simulink model "dgbe_test"  (Simulink 7.4)
settings: Solver=ode45  StartTime=0.0  StopTime=10.0  RelTol=1e-3
undefined symbols (not defined in the file or in its folder): ROACH
libraries: xbsIndex_r4 x109, xps_library x27
settings Model: Creator=tfiliba  LastModifiedBy=tfiliba

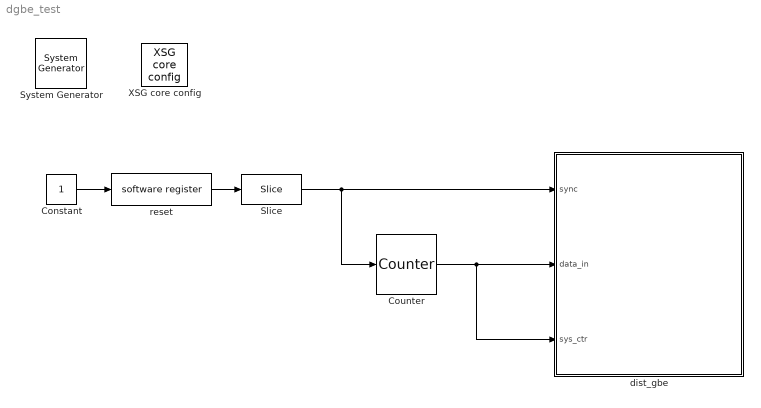
== system dgbe_test ==
  " System Generator" : xbsIndex_r4/ System Generator  Tag=genX  SystemSampleTime=-1  xilinxfamily=virtex5  part=xc5vsx95t  speed=-1  package=ff1136  synthesis_tool=XST  clock_wrapper=Clock Enables  directory=./dgbe_test/sysgen  testbench=off  simulink_period=1  sysclk_period=3.9062  dcm_input_clock_period=100  incr_netlist=off  trim_vbits=Everywhere in SubSystem  dbl_ovrd=According to Block Masks  core_generation=According to Block Masks  run_coregen=off  deprecated_control=off  eval_field=0  block_type=sysgen
      settings: block_version=11.4
  Constant : Constant  OutDataType=fixdt(1, 16)  OutScaling=2^0
  Counter : xbsIndex_r4/Counter  cnt_type=Free Running  cnt_to=Inf  operation=Up  start_count=0  cnt_by_val=1  arith_type=Unsigned  n_bits=64  bin_pt=0  load_pin=off  rst=on  en=off  explicit_period=on  period=1  dbl_ovrd=off  use_behavioral_HDL=off  implementation=Fabric  block_type=counter
      settings: block_version=11.4
  Slice : xbsIndex_r4/Slice  nbits=1  boolean_output=on  mode=Upper Bit Location + Width  bit1=0  base1=MSB of Input  bit0=0  base0=LSB of Input  dbl_ovrd=off  block_type=slice
  XSG core config : xps_library/XSG core config  Tag=xps:xsg  SystemSampleTime=-1  hw_sys=ROACH:sx95t  ibob_linux=off  clk_src=aux0_clk  iBOB_clk_src=sys_clk  BEE2_ctrl_clk_src=sys_clk  BEE2_usr_clk_src=sys_clk  ROACH_clk_src=aux0_clk  CORR_clk_src=sys_clk  gpio_clk_io_group=iBOB:sma  gpio_clk_bit_index=0  clk_rate=256  sample_period=1  synthesis_tool=XST  mpc_type=powerpc440_ext
  dist_gbe : Subsystem  mask(dist_gbe){numcomputers=8, samplesperpacket=1024, numtengbe=4}
      mask prompts: numcomputers "Num IPs (Must be power of 2)"; samplesperpacket "Samples per packet (Number of samples to put in a packet)"; numtengbe "Number of tengbe ports"
      mask init:
      | cfg.source = str2func('dist_gbe_xblock_init');
      | cfg.toplevel = gcb;
      | cfg.depend = {'dist_gbe_xblock_init.m'};
      | args = {numcomputers,samplesperpacket,numtengbe};
      | xBlock(cfg, args);
  reset : xps_library/software register  Tag=xps:sw_reg  SystemSampleTime=-1  io_dir=From Processor  arith_type=Unsigned  bitwidth=32  bin_pt=0  sample_period=1  gw_name=dgbe_test_reset_user_data_out
  wires:
  Constant/1 -> reset/1
  Counter/1 -> dist_gbe/2(data_in), dist_gbe/3(sys_ctr)
  reset/1 -> Slice/1
  Slice/1 -> Counter/1, dist_gbe/1(sync)

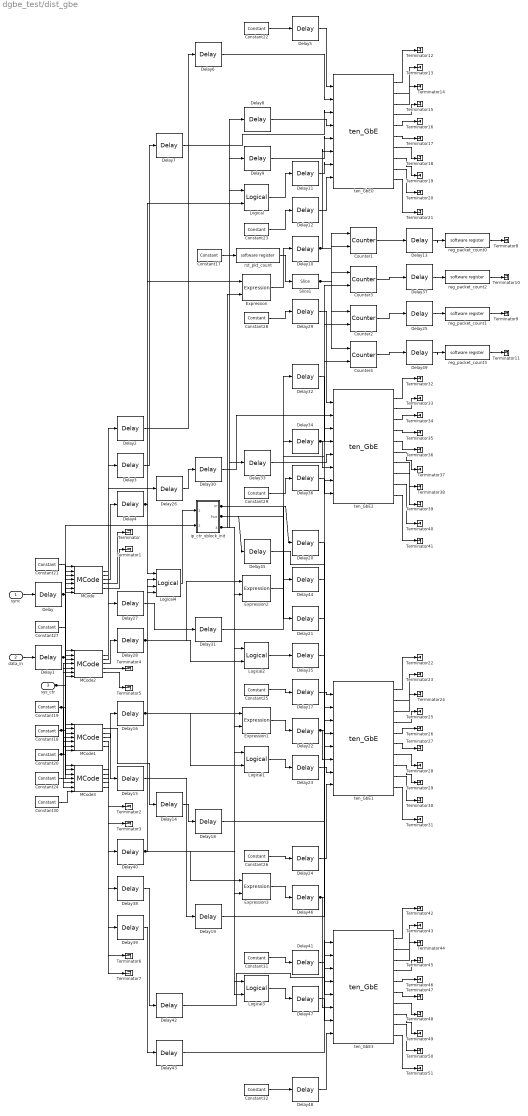
== system dgbe_test/dist_gbe ==
  sync : Inport
  data_in : Inport  Port=2
  sys_ctr : Inport  Port=3
  Constant17 : xbsIndex_r4/Constant  arith_type=Signed (2's comp)  const=0  n_bits=16  bin_pt=14  explicit_period=on  period=1  equ=P=C  opselect=C  inp2=PCIN>>17  opr=+  inp1=P  carry=CIN  dbl_ovrd=off  block_type=constant
      settings: block_version=11.4
  Constant18 : xbsIndex_r4/Constant  arith_type=Signed (2's comp)  const=8  n_bits=4  bin_pt=0  explicit_period=on  period=1  equ=P=C  opselect=C  inp2=PCIN>>17  opr=+  inp1=P  carry=CIN  dbl_ovrd=off  block_type=constant
      settings: block_version=11.4
  Constant19 : xbsIndex_r4/Constant  arith_type=Signed (2's comp)  const=1024  n_bits=11  bin_pt=0  explicit_period=on  period=1  equ=P=C  opselect=C  inp2=PCIN>>17  opr=+  inp1=P  carry=CIN  dbl_ovrd=off  block_type=constant
      settings: block_version=11.4
  Constant20 : xbsIndex_r4/Constant  arith_type=Signed (2's comp)  const=4  n_bits=3  bin_pt=0  explicit_period=on  period=1  equ=P=C  opselect=C  inp2=PCIN>>17  opr=+  inp1=P  carry=CIN  dbl_ovrd=off  block_type=constant
      settings: block_version=11.4
  Constant21 : xbsIndex_r4/Constant  arith_type=Signed (2's comp)  const=0  n_bits=3  bin_pt=0  explicit_period=on  period=1  equ=P=C  opselect=C  inp2=PCIN>>17  opr=+  inp1=P  carry=CIN  dbl_ovrd=off  block_type=constant
      settings: block_version=11.4
  Constant{22..23,25..26,28..29,31..32} (8 alike) : xbsIndex_r4/Constant  arith_type=Boolean  const=0  n_bits=16  bin_pt=14  explicit_period=on  period=1  equ=P=C  opselect=C  inp2=PCIN>>17  opr=+  inp1=P  carry=CIN  dbl_ovrd=off  block_type=constant
      settings: block_version=11.4
  Constant24 : xbsIndex_r4/Constant  arith_type=Signed (2's comp)  const=1  n_bits=3  bin_pt=0  explicit_period=on  period=1  equ=P=C  opselect=C  inp2=PCIN>>17  opr=+  inp1=P  carry=CIN  dbl_ovrd=off  block_type=constant
      settings: block_version=11.4
  Constant27 : xbsIndex_r4/Constant  arith_type=Signed (2's comp)  const=2  n_bits=3  bin_pt=0  explicit_period=on  period=1  equ=P=C  opselect=C  inp2=PCIN>>17  opr=+  inp1=P  carry=CIN  dbl_ovrd=off  block_type=constant
      settings: block_version=11.4
  Constant30 : xbsIndex_r4/Constant  arith_type=Signed (2's comp)  const=3  n_bits=3  bin_pt=0  explicit_period=on  period=1  equ=P=C  opselect=C  inp2=PCIN>>17  opr=+  inp1=P  carry=CIN  dbl_ovrd=off  block_type=constant
      settings: block_version=11.4
  Counter{1..4} (4 alike) : xbsIndex_r4/Counter  cnt_type=Free Running  cnt_to=Inf  operation=Up  start_count=0  cnt_by_val=1  arith_type=Unsigned  n_bits=32  bin_pt=0  load_pin=off  rst=on  en=on  explicit_period=on  period=1  dbl_ovrd=off  use_behavioral_HDL=off  implementation=Fabric  block_type=counter
      settings: block_version=11.4
  Delay : xbsIndex_r4/Delay  en=off  latency=3  dbl_ovrd=off  reg_retiming=on  block_type=delay
      settings: block_version=11.4
  Delay1 : xbsIndex_r4/Delay  en=off  latency=3  dbl_ovrd=off  reg_retiming=on  block_type=delay
      settings: block_version=11.4
  Delay{2..49} (48 alike) : xbsIndex_r4/Delay  en=off  latency=2  dbl_ovrd=off  reg_retiming=on  block_type=delay
      settings: block_version=11.4
  Expression{,1..3} (4 alike) : xbsIndex_r4/Expression  expression=a&~b  align_bp=on  en=off  latency=0  precision=Full  arith_type=Unsigned  n_bits=16  bin_pt=0  dbl_ovrd=off  block_type=expr
      settings: block_version=11.4
  Logical{,1..3} (4 alike) : xbsIndex_r4/Logical  logical_function=AND  inputs=2  en=off  latency=0  precision=Full  arith_type=Unsigned  n_bits=16  bin_pt=0  align_bp=on  dbl_ovrd=off  block_type=logical
      settings: block_version=11.4
  Logical4 : xbsIndex_r4/Logical  logical_function=OR  inputs=4  en=off  latency=0  precision=Full  arith_type=Unsigned  n_bits=16  bin_pt=0  align_bp=on  dbl_ovrd=off  block_type=logical
      settings: block_version=11.4
  MCode{,1..3} (4 alike) : xbsIndex_r4/MCode  mfname=packetizer.m  explicit_period=off  period=1  dbl_ovrd=off  enable_stdout=off  enable_debug=off  suppress_output=on  defparams={}  hide_port_list={}  block_type=mcode
      settings: block_version=11.4
  Slice1 : xbsIndex_r4/Slice  nbits=1  boolean_output=on  mode=Upper Bit Location + Width  bit1=0  base1=MSB of Input  bit0=0  base0=LSB of Input  dbl_ovrd=off  block_type=slice
  Terminator{,1..51} (52 alike) : Terminator
  ip_ctr_xblock_init : Subsystem
  reg_packet_count0 : xps_library/software register  Tag=xps:sw_reg  SystemSampleTime=-1  io_dir=To Processor  arith_type=Unsigned  bitwidth=32  bin_pt=0  sample_period=1  gw_name=dgbe_test_dist_gbe_reg_packet_count0_user_data_in
  reg_packet_count1 : xps_library/software register  Tag=xps:sw_reg  SystemSampleTime=-1  io_dir=To Processor  arith_type=Unsigned  bitwidth=32  bin_pt=0  sample_period=1  gw_name=dgbe_test_dist_gbe_reg_packet_count1_user_data_in
  reg_packet_count2 : xps_library/software register  Tag=xps:sw_reg  SystemSampleTime=-1  io_dir=To Processor  arith_type=Unsigned  bitwidth=32  bin_pt=0  sample_period=1  gw_name=dgbe_test_dist_gbe_reg_packet_count2_user_data_in
  reg_packet_count3 : xps_library/software register  Tag=xps:sw_reg  SystemSampleTime=-1  io_dir=To Processor  arith_type=Unsigned  bitwidth=32  bin_pt=0  sample_period=1  gw_name=dgbe_test_dist_gbe_reg_packet_count3_user_data_in
  rst_pkt_count : xps_library/software register  Tag=xps:sw_reg  SystemSampleTime=-1  io_dir=From Processor  arith_type=Unsigned  bitwidth=32  bin_pt=0  sample_period=1  gw_name=dgbe_test_dist_gbe_rst_pkt_count_user_data_out
  ten_GbE0 : xps_library/ten_GbE  Tag=xps:tengbe  SystemSampleTime=-1  port=ROACH:0  mac_lite=off  open_phy=off  show_param=off  pre_emph=3  swing=800  fab_en=off  fab_mac=0  fab_ip=0  fab_udp=0  fab_gate=0
  ten_GbE1 : xps_library/ten_GbE  Tag=xps:tengbe  SystemSampleTime=-1  port=ROACH:1  mac_lite=off  open_phy=off  show_param=off  pre_emph=3  swing=800  fab_en=off  fab_mac=0  fab_ip=0  fab_udp=0  fab_gate=0
  ten_GbE2 : xps_library/ten_GbE  Tag=xps:tengbe  SystemSampleTime=-1  port=ROACH:2  mac_lite=off  open_phy=off  show_param=off  pre_emph=3  swing=800  fab_en=off  fab_mac=0  fab_ip=0  fab_udp=0  fab_gate=0
  ten_GbE3 : xps_library/ten_GbE  Tag=xps:tengbe  SystemSampleTime=-1  port=ROACH:3  mac_lite=off  open_phy=off  show_param=off  pre_emph=3  swing=800  fab_en=off  fab_mac=0  fab_ip=0  fab_udp=0  fab_gate=0
  wires:
  Delay/1 -> MCode3/1, MCode2/1, MCode1/1, MCode/1, ip_ctr_xblock_init/2(Reset)
  Delay1/1 -> MCode3/2, MCode2/2, MCode1/2, MCode/2
  sys_ctr/1 -> MCode3/3, MCode2/3, MCode1/3, MCode/3
  Constant19/1 -> MCode3/4, MCode2/4, MCode1/4, MCode/4
  Constant18/1 -> MCode3/5, MCode2/5, MCode1/5, MCode/5
  Constant20/1 -> MCode3/6, MCode2/6, MCode1/6, MCode/6
  Delay4/1 -> Logical4/1, Logical/2, Expression/1
  ip_ctr_xblock_init/3(Discard_pkt) -> Logical3/1, Expression3/2, Logical2/1, Expression2/2, Logical1/1, Expression1/2, Logical/1, Expression/2
  ip_ctr_xblock_init/1(IP) -> Delay44/1, Delay32/1, Delay20/1, Delay8/1
  ip_ctr_xblock_init/2(Port) -> Delay45/1, Delay33/1, Delay21/1, Delay9/1
  Delay10/1 -> Counter1/2, ten_GbE0/6
  Slice1/1 -> Counter4/1, Counter3/1, Counter2/1, Counter1/1
  Delay16/1 -> Logical4/2, Logical1/2, Expression1/1
  Delay22/1 -> Counter2/2, ten_GbE1/6
  Delay28/1 -> Logical4/3, Logical2/2, Expression2/1
  Delay34/1 -> Counter3/2, ten_GbE2/6
  Delay40/1 -> Logical4/4, Logical3/2, Expression3/1
  Delay46/1 -> Counter4/2, ten_GbE3/6
  ten_GbE3/10 -> Terminator51/1
  ten_GbE3/9 -> Terminator50/1
  ten_GbE3/8 -> Terminator49/1
  ten_GbE3/7 -> Terminator48/1
  ten_GbE3/6 -> Terminator47/1
  ten_GbE3/5 -> Terminator46/1
  ten_GbE3/4 -> Terminator45/1
  ten_GbE3/3 -> Terminator44/1
  ten_GbE3/2 -> Terminator43/1
  ten_GbE3/1 -> Terminator42/1
  ten_GbE2/10 -> Terminator41/1
  ten_GbE2/9 -> Terminator40/1
  ten_GbE2/8 -> Terminator39/1
  ten_GbE2/7 -> Terminator38/1
  ten_GbE2/6 -> Terminator37/1
  ten_GbE2/5 -> Terminator36/1
  ten_GbE2/4 -> Terminator35/1
  ten_GbE2/3 -> Terminator34/1
  ten_GbE2/2 -> Terminator33/1
  ten_GbE2/1 -> Terminator32/1
  ten_GbE1/10 -> Terminator31/1
  ten_GbE1/9 -> Terminator30/1
  ten_GbE1/8 -> Terminator29/1
  ten_GbE1/7 -> Terminator28/1
  ten_GbE1/6 -> Terminator27/1
  ten_GbE1/5 -> Terminator26/1
  ten_GbE1/4 -> Terminator25/1
  ten_GbE1/3 -> Terminator24/1
  ten_GbE1/2 -> Terminator23/1
  ten_GbE1/1 -> Terminator22/1
  ten_GbE0/10 -> Terminator21/1
  ten_GbE0/9 -> Terminator20/1
  ten_GbE0/8 -> Terminator19/1
  ten_GbE0/7 -> Terminator18/1
  ten_GbE0/6 -> Terminator17/1
  ten_GbE0/5 -> Terminator16/1
  ten_GbE0/4 -> Terminator15/1
  ten_GbE0/3 -> Terminator14/1
  ten_GbE0/2 -> Terminator13/1
  ten_GbE0/1 -> Terminator12/1
  reg_packet_count3/1 -> Terminator11/1
  reg_packet_count2/1 -> Terminator10/1
  reg_packet_count1/1 -> Terminator9/1
  reg_packet_count0/1 -> Terminator8/1
  MCode3/5 -> Terminator7/1
  MCode3/4 -> Terminator6/1
  MCode2/5 -> Terminator5/1
  MCode2/4 -> Terminator4/1
  MCode1/5 -> Terminator3/1
  MCode1/4 -> Terminator2/1
  MCode/5 -> Terminator1/1
  MCode/4 -> Terminator/1
  Logical4/1 -> ip_ctr_xblock_init/1(Count)
  Delay49/1 -> reg_packet_count3/1
  Counter4/1 -> Delay49/1
  Delay48/1 -> ten_GbE3/8
  Delay47/1 -> ten_GbE3/7
  Delay45/1 -> ten_GbE3/5
  Delay44/1 -> ten_GbE3/4
  Delay43/1 -> ten_GbE3/3
  Delay42/1 -> ten_GbE3/2
  Delay41/1 -> ten_GbE3/1
  Constant32/1 -> Delay48/1
  Logical3/1 -> Delay47/1
  Expression3/1 -> Delay46/1
  Delay39/1 -> Delay43/1
  Delay38/1 -> Delay42/1
  Constant31/1 -> Delay41/1
  MCode3/3 -> Delay40/1
  MCode3/2 -> Delay39/1
  MCode3/1 -> Delay38/1
  Constant30/1 -> MCode3/7
  Delay37/1 -> reg_packet_count2/1
  Counter3/1 -> Delay37/1
  Delay36/1 -> ten_GbE2/8
  Delay35/1 -> ten_GbE2/7
  Delay33/1 -> ten_GbE2/5
  Delay32/1 -> ten_GbE2/4
  Delay31/1 -> ten_GbE2/3
  Delay30/1 -> ten_GbE2/2
  Delay29/1 -> ten_GbE2/1
  Constant29/1 -> Delay36/1
  Logical2/1 -> Delay35/1
  Expression2/1 -> Delay34/1
  Delay27/1 -> Delay31/1
  Delay26/1 -> Delay30/1
  Constant28/1 -> Delay29/1
  MCode2/3 -> Delay28/1
  MCode2/2 -> Delay27/1
  MCode2/1 -> Delay26/1
  Constant27/1 -> MCode2/7
  Delay25/1 -> reg_packet_count1/1
  Counter2/1 -> Delay25/1
  Delay24/1 -> ten_GbE1/8
  Delay23/1 -> ten_GbE1/7
  Delay21/1 -> ten_GbE1/5
  Delay20/1 -> ten_GbE1/4
  Delay19/1 -> ten_GbE1/3
  Delay18/1 -> ten_GbE1/2
  Delay17/1 -> ten_GbE1/1
  Constant26/1 -> Delay24/1
  Logical1/1 -> Delay23/1
  Expression1/1 -> Delay22/1
  Delay15/1 -> Delay19/1
  Delay14/1 -> Delay18/1
  Constant25/1 -> Delay17/1
  MCode1/3 -> Delay16/1
  MCode1/2 -> Delay15/1
  MCode1/1 -> Delay14/1
  Constant24/1 -> MCode1/7
  Delay13/1 -> reg_packet_count0/1
  Counter1/1 -> Delay13/1
  Delay12/1 -> ten_GbE0/8
  Delay11/1 -> ten_GbE0/7
  Delay9/1 -> ten_GbE0/5
  Delay8/1 -> ten_GbE0/4
  Delay7/1 -> ten_GbE0/3
  Delay6/1 -> ten_GbE0/2
  Delay5/1 -> ten_GbE0/1
  Constant23/1 -> Delay12/1
  Logical/1 -> Delay11/1
  Expression/1 -> Delay10/1
  Delay3/1 -> Delay7/1
  Delay2/1 -> Delay6/1
  Constant22/1 -> Delay5/1
  MCode/3 -> Delay4/1
  MCode/2 -> Delay3/1
  MCode/1 -> Delay2/1
  Constant21/1 -> MCode/7
  rst_pkt_count/1 -> Slice1/1
  Constant17/1 -> rst_pkt_count/1
  data_in/1 -> Delay1/1
  sync/1 -> Delay/1

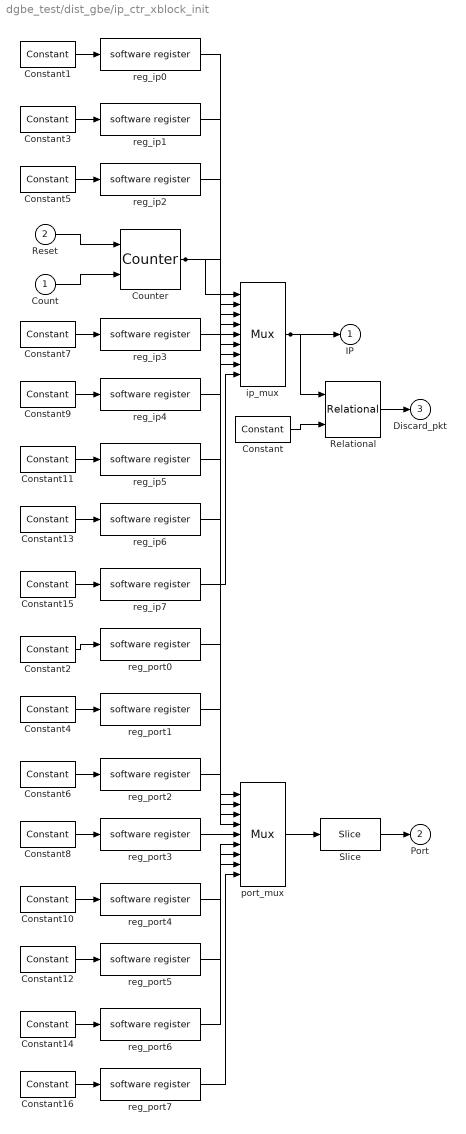
== system dgbe_test/dist_gbe/ip_ctr_xblock_init ==
  Count : Inport
  Reset : Inport  Port=2
  Constant : xbsIndex_r4/Constant  arith_type=Unsigned  const=0  n_bits=32  bin_pt=0  explicit_period=on  period=1  equ=P=C  opselect=C  inp2=PCIN>>17  opr=+  inp1=P  carry=CIN  dbl_ovrd=off  block_type=constant
      settings: block_version=11.4
  Constant1 : xbsIndex_r4/Constant  arith_type=Signed (2's comp)  const=4001  n_bits=16  bin_pt=0  explicit_period=on  period=1  equ=P=C  opselect=C  inp2=PCIN>>17  opr=+  inp1=P  carry=CIN  dbl_ovrd=off  block_type=constant
      settings: block_version=11.4
  Constant10 : xbsIndex_r4/Constant  arith_type=Signed (2's comp)  const=4005  n_bits=16  bin_pt=0  explicit_period=on  period=1  equ=P=C  opselect=C  inp2=PCIN>>17  opr=+  inp1=P  carry=CIN  dbl_ovrd=off  block_type=constant
      settings: block_version=11.4
  Constant11 : xbsIndex_r4/Constant  arith_type=Signed (2's comp)  const=4006  n_bits=16  bin_pt=0  explicit_period=on  period=1  equ=P=C  opselect=C  inp2=PCIN>>17  opr=+  inp1=P  carry=CIN  dbl_ovrd=off  block_type=constant
      settings: block_version=11.4
  Constant12 : xbsIndex_r4/Constant  arith_type=Signed (2's comp)  const=4006  n_bits=16  bin_pt=0  explicit_period=on  period=1  equ=P=C  opselect=C  inp2=PCIN>>17  opr=+  inp1=P  carry=CIN  dbl_ovrd=off  block_type=constant
      settings: block_version=11.4
  Constant13 : xbsIndex_r4/Constant  arith_type=Signed (2's comp)  const=4007  n_bits=16  bin_pt=0  explicit_period=on  period=1  equ=P=C  opselect=C  inp2=PCIN>>17  opr=+  inp1=P  carry=CIN  dbl_ovrd=off  block_type=constant
      settings: block_version=11.4
  Constant14 : xbsIndex_r4/Constant  arith_type=Signed (2's comp)  const=4007  n_bits=16  bin_pt=0  explicit_period=on  period=1  equ=P=C  opselect=C  inp2=PCIN>>17  opr=+  inp1=P  carry=CIN  dbl_ovrd=off  block_type=constant
      settings: block_version=11.4
  Constant15 : xbsIndex_r4/Constant  arith_type=Signed (2's comp)  const=4008  n_bits=16  bin_pt=0  explicit_period=on  period=1  equ=P=C  opselect=C  inp2=PCIN>>17  opr=+  inp1=P  carry=CIN  dbl_ovrd=off  block_type=constant
      settings: block_version=11.4
  Constant16 : xbsIndex_r4/Constant  arith_type=Signed (2's comp)  const=4008  n_bits=16  bin_pt=0  explicit_period=on  period=1  equ=P=C  opselect=C  inp2=PCIN>>17  opr=+  inp1=P  carry=CIN  dbl_ovrd=off  block_type=constant
      settings: block_version=11.4
  Constant2 : xbsIndex_r4/Constant  arith_type=Signed (2's comp)  const=4001  n_bits=16  bin_pt=0  explicit_period=on  period=1  equ=P=C  opselect=C  inp2=PCIN>>17  opr=+  inp1=P  carry=CIN  dbl_ovrd=off  block_type=constant
      settings: block_version=11.4
  Constant3 : xbsIndex_r4/Constant  arith_type=Signed (2's comp)  const=4002  n_bits=16  bin_pt=0  explicit_period=on  period=1  equ=P=C  opselect=C  inp2=PCIN>>17  opr=+  inp1=P  carry=CIN  dbl_ovrd=off  block_type=constant
      settings: block_version=11.4
  Constant4 : xbsIndex_r4/Constant  arith_type=Signed (2's comp)  const=4002  n_bits=16  bin_pt=0  explicit_period=on  period=1  equ=P=C  opselect=C  inp2=PCIN>>17  opr=+  inp1=P  carry=CIN  dbl_ovrd=off  block_type=constant
      settings: block_version=11.4
  Constant5 : xbsIndex_r4/Constant  arith_type=Signed (2's comp)  const=4003  n_bits=16  bin_pt=0  explicit_period=on  period=1  equ=P=C  opselect=C  inp2=PCIN>>17  opr=+  inp1=P  carry=CIN  dbl_ovrd=off  block_type=constant
      settings: block_version=11.4
  Constant6 : xbsIndex_r4/Constant  arith_type=Signed (2's comp)  const=4003  n_bits=16  bin_pt=0  explicit_period=on  period=1  equ=P=C  opselect=C  inp2=PCIN>>17  opr=+  inp1=P  carry=CIN  dbl_ovrd=off  block_type=constant
      settings: block_version=11.4
  Constant7 : xbsIndex_r4/Constant  arith_type=Signed (2's comp)  const=4004  n_bits=16  bin_pt=0  explicit_period=on  period=1  equ=P=C  opselect=C  inp2=PCIN>>17  opr=+  inp1=P  carry=CIN  dbl_ovrd=off  block_type=constant
      settings: block_version=11.4
  Constant8 : xbsIndex_r4/Constant  arith_type=Signed (2's comp)  const=4004  n_bits=16  bin_pt=0  explicit_period=on  period=1  equ=P=C  opselect=C  inp2=PCIN>>17  opr=+  inp1=P  carry=CIN  dbl_ovrd=off  block_type=constant
      settings: block_version=11.4
  Constant9 : xbsIndex_r4/Constant  arith_type=Signed (2's comp)  const=4005  n_bits=16  bin_pt=0  explicit_period=on  period=1  equ=P=C  opselect=C  inp2=PCIN>>17  opr=+  inp1=P  carry=CIN  dbl_ovrd=off  block_type=constant
      settings: block_version=11.4
  Counter : xbsIndex_r4/Counter  cnt_type=Free Running  cnt_to=Inf  operation=Up  start_count=0  cnt_by_val=1  arith_type=Unsigned  n_bits=3  bin_pt=0  load_pin=off  rst=on  en=on  explicit_period=on  period=1  dbl_ovrd=off  use_behavioral_HDL=off  implementation=Fabric  block_type=counter
      settings: block_version=11.4
  Relational : xbsIndex_r4/Relational  mode=a=b  en=off  latency=1  dbl_ovrd=off  block_type=relational
  Slice : xbsIndex_r4/Slice  nbits=16  boolean_output=off  mode=Lower Bit Location + Width  bit1=0  base1=MSB of Input  bit0=0  base0=LSB of Input  dbl_ovrd=off  block_type=slice
  ip_mux : xbsIndex_r4/Mux  inputs=8  en=off  latency=3  precision=Full  arith_type=Unsigned  n_bits=16  bin_pt=14  quantization=Truncate  overflow=Wrap  dbl_ovrd=off  block_type=mux
      settings: block_version=11.4
  port_mux : xbsIndex_r4/Mux  inputs=8  en=off  latency=3  precision=Full  arith_type=Unsigned  n_bits=16  bin_pt=14  quantization=Truncate  overflow=Wrap  dbl_ovrd=off  block_type=mux
      settings: block_version=11.4
  reg_ip0 : xps_library/software register  Tag=xps:sw_reg  SystemSampleTime=-1  io_dir=From Processor  arith_type=Unsigned  bitwidth=32  bin_pt=0  sample_period=1  gw_name=dgbe_test_dist_gbe_ip_ctr_xblock_init_reg_ip0_user_data_out
  reg_ip1 : xps_library/software register  Tag=xps:sw_reg  SystemSampleTime=-1  io_dir=From Processor  arith_type=Unsigned  bitwidth=32  bin_pt=0  sample_period=1  gw_name=dgbe_test_dist_gbe_ip_ctr_xblock_init_reg_ip1_user_data_out
  reg_ip2 : xps_library/software register  Tag=xps:sw_reg  SystemSampleTime=-1  io_dir=From Processor  arith_type=Unsigned  bitwidth=32  bin_pt=0  sample_period=1  gw_name=dgbe_test_dist_gbe_ip_ctr_xblock_init_reg_ip2_user_data_out
  reg_ip3 : xps_library/software register  Tag=xps:sw_reg  SystemSampleTime=-1  io_dir=From Processor  arith_type=Unsigned  bitwidth=32  bin_pt=0  sample_period=1  gw_name=dgbe_test_dist_gbe_ip_ctr_xblock_init_reg_ip3_user_data_out
  reg_ip4 : xps_library/software register  Tag=xps:sw_reg  SystemSampleTime=-1  io_dir=From Processor  arith_type=Unsigned  bitwidth=32  bin_pt=0  sample_period=1  gw_name=dgbe_test_dist_gbe_ip_ctr_xblock_init_reg_ip4_user_data_out
  reg_ip5 : xps_library/software register  Tag=xps:sw_reg  SystemSampleTime=-1  io_dir=From Processor  arith_type=Unsigned  bitwidth=32  bin_pt=0  sample_period=1  gw_name=dgbe_test_dist_gbe_ip_ctr_xblock_init_reg_ip5_user_data_out
  reg_ip6 : xps_library/software register  Tag=xps:sw_reg  SystemSampleTime=-1  io_dir=From Processor  arith_type=Unsigned  bitwidth=32  bin_pt=0  sample_period=1  gw_name=dgbe_test_dist_gbe_ip_ctr_xblock_init_reg_ip6_user_data_out
  reg_ip7 : xps_library/software register  Tag=xps:sw_reg  SystemSampleTime=-1  io_dir=From Processor  arith_type=Unsigned  bitwidth=32  bin_pt=0  sample_period=1  gw_name=dgbe_test_dist_gbe_ip_ctr_xblock_init_reg_ip7_user_data_out
  reg_port0 : xps_library/software register  Tag=xps:sw_reg  SystemSampleTime=-1  io_dir=From Processor  arith_type=Unsigned  bitwidth=32  bin_pt=0  sample_period=1  gw_name=dgbe_test_dist_gbe_ip_ctr_xblock_init_reg_port0_user_data_out
  reg_port1 : xps_library/software register  Tag=xps:sw_reg  SystemSampleTime=-1  io_dir=From Processor  arith_type=Unsigned  bitwidth=32  bin_pt=0  sample_period=1  gw_name=dgbe_test_dist_gbe_ip_ctr_xblock_init_reg_port1_user_data_out
  reg_port2 : xps_library/software register  Tag=xps:sw_reg  SystemSampleTime=-1  io_dir=From Processor  arith_type=Unsigned  bitwidth=32  bin_pt=0  sample_period=1  gw_name=dgbe_test_dist_gbe_ip_ctr_xblock_init_reg_port2_user_data_out
  reg_port3 : xps_library/software register  Tag=xps:sw_reg  SystemSampleTime=-1  io_dir=From Processor  arith_type=Unsigned  bitwidth=32  bin_pt=0  sample_period=1  gw_name=dgbe_test_dist_gbe_ip_ctr_xblock_init_reg_port3_user_data_out
  reg_port4 : xps_library/software register  Tag=xps:sw_reg  SystemSampleTime=-1  io_dir=From Processor  arith_type=Unsigned  bitwidth=32  bin_pt=0  sample_period=1  gw_name=dgbe_test_dist_gbe_ip_ctr_xblock_init_reg_port4_user_data_out
  reg_port5 : xps_library/software register  Tag=xps:sw_reg  SystemSampleTime=-1  io_dir=From Processor  arith_type=Unsigned  bitwidth=32  bin_pt=0  sample_period=1  gw_name=dgbe_test_dist_gbe_ip_ctr_xblock_init_reg_port5_user_data_out
  reg_port6 : xps_library/software register  Tag=xps:sw_reg  SystemSampleTime=-1  io_dir=From Processor  arith_type=Unsigned  bitwidth=32  bin_pt=0  sample_period=1  gw_name=dgbe_test_dist_gbe_ip_ctr_xblock_init_reg_port6_user_data_out
  reg_port7 : xps_library/software register  Tag=xps:sw_reg  SystemSampleTime=-1  io_dir=From Processor  arith_type=Unsigned  bitwidth=32  bin_pt=0  sample_period=1  gw_name=dgbe_test_dist_gbe_ip_ctr_xblock_init_reg_port7_user_data_out
  IP : Outport
  Port : Outport  Port=2
  Discard_pkt : Outport  Port=3
  wires:
  Counter/1 -> port_mux/1, ip_mux/1
  ip_mux/1 -> Relational/1, IP/1
  port_mux/1 -> Slice/1
  reg_port7/1 -> port_mux/9
  reg_port6/1 -> port_mux/8
  reg_port5/1 -> port_mux/7
  reg_port4/1 -> port_mux/6
  reg_port3/1 -> port_mux/5
  reg_port2/1 -> port_mux/4
  reg_port1/1 -> port_mux/3
  reg_port0/1 -> port_mux/2
  reg_ip7/1 -> ip_mux/9
  reg_ip6/1 -> ip_mux/8
  reg_ip5/1 -> ip_mux/7
  reg_ip4/1 -> ip_mux/6
  reg_ip3/1 -> ip_mux/5
  reg_ip2/1 -> ip_mux/4
  reg_ip1/1 -> ip_mux/3
  reg_ip0/1 -> ip_mux/2
  Constant16/1 -> reg_port7/1
  Constant15/1 -> reg_ip7/1
  Constant14/1 -> reg_port6/1
  Constant13/1 -> reg_ip6/1
  Constant12/1 -> reg_port5/1
  Constant11/1 -> reg_ip5/1
  Constant10/1 -> reg_port4/1
  Constant9/1 -> reg_ip4/1
  Constant8/1 -> reg_port3/1
  Constant7/1 -> reg_ip3/1
  Constant6/1 -> reg_port2/1
  Constant5/1 -> reg_ip2/1
  Constant4/1 -> reg_port1/1
  Constant3/1 -> reg_ip1/1
  Constant2/1 -> reg_port0/1
  Constant1/1 -> reg_ip0/1
  Relational/1 -> Discard_pkt/1
  Constant/1 -> Relational/2
  Count/1 -> Counter/2
  Reset/1 -> Counter/1
  Slice/1 -> Port/1
